simulink model "Hibrida_ultima"  (R2021b)
settings: Solver=VariableStepAuto  StartTime=0.0  StopTime=10.0  RelTol=1e-3
PreLoadFcn:
  | Fs = 44100;
  | f_tono = 500;
  | L = 32;
InitFcn:
  | Fs = 44100;
  | f_tono = 500;
  | L = 32;
undefined symbols (not defined in the file or in its folder): SzEstimado
settings Model: Creator=Vale Oieni  LastModifiedBy=ValeOieni

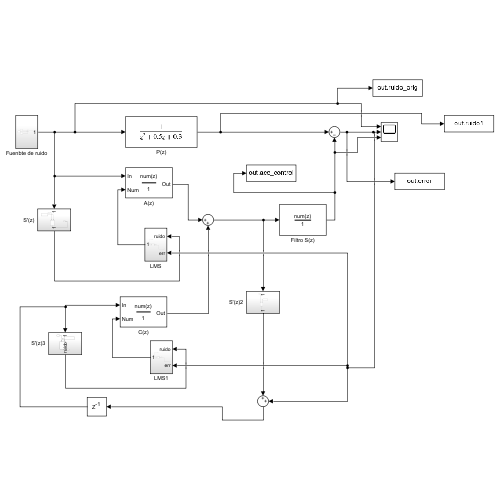
[thumbnail: Simulink's stored preview of the top-level diagram]
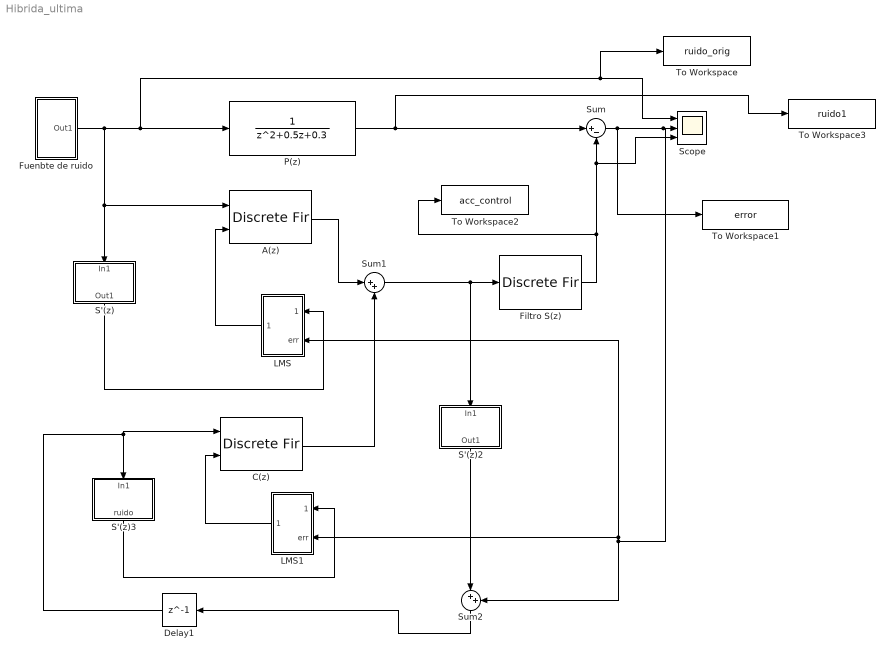
== system Hibrida_ultima ==
  A(z) : DiscreteFir  CoefSource=Input port  SampleTime=1/Fs
      settings: InputPortMap=u0,u1
  C(z) : DiscreteFir  CoefSource=Input port  SampleTime=1/Fs
      settings: InputPortMap=u0,u1
  Delay1 : Delay  DelayLength=1  InitialCondition=0
  Filtro S(z) : DiscreteFir  Coefficients=[0 0 -.5 .5 -.3 .2 -.1 .5 -.5]  InputProcessing=Columns as channels (frame based)  SampleTime=1/Fs
  Fuenbte de ruido : Subsystem
  LMS : Subsystem
  LMS1 : Subsystem
  P(z) : DiscreteTransferFcn  Denominator="[1 0.5  0.3]"
  S'(z) : Subsystem
  S'(z)2 : Subsystem
  S'(z)3 : Subsystem
  Scope : Scope  NumInputPorts=3
  Sum : Sum  Inputs=|+-
  Sum1 : Sum  Inputs=|++
  Sum2 : Sum  Inputs=|++
  To Workspace : ToWorkspace  VariableName=ruido_orig  SampleTime=-1
      settings: Save2DSignal=2-D array (concatenate along first dimension)
  To Workspace1 : ToWorkspace  VariableName=error  SampleTime=-1
      settings: Save2DSignal=2-D array (concatenate along first dimension)
  To Workspace2 : ToWorkspace  VariableName=acc_control  SampleTime=-1
      settings: Save2DSignal=2-D array (concatenate along first dimension)
  To Workspace3 : ToWorkspace  VariableName=ruido1  SampleTime=-1
      settings: Save2DSignal=2-D array (concatenate along first dimension)
  wires:
  Fuenbte de ruido/1(Out1) -> To Workspace/1, Scope/1, P(z)/1, A(z)/1, S'(z)/1(In1)
  P(z)/1 -> To Workspace3/1, Sum/1
  Filtro S(z)/1 -> Scope/3, Sum/2, To Workspace2/1
  Sum/1 -> To Workspace1/1, LMS1/2(err), LMS/2(err), Sum2/2, Scope/2
  Sum1/1 -> Filtro S(z)/1, S'(z)2/1(In1)
  A(z)/1 -> Sum1/1
  C(z)/1 -> Sum1/2
  LMS/1(Out1) -> A(z)/2
  LMS1/1(Out1) -> C(z)/2
  Sum2/1 -> Delay1/1
  S'(z)3/1(ruido) -> LMS1/1(ruido)
  S'(z)/1(Out1) -> LMS/1(ruido)
  S'(z)2/1(Out1) -> Sum2/1
  Delay1/1 -> C(z)/1, S'(z)3/1(In1)

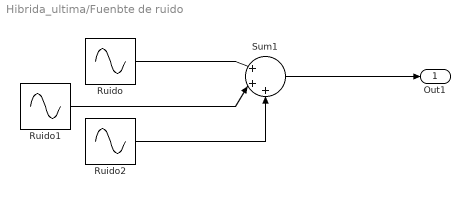
== system Hibrida_ultima/Fuenbte de ruido ==
  Ruido : Sin  Frequency=f_tono*(2*pi)  SampleTime=1/Fs
  Ruido1 : Sin  Frequency=2*f_tono*(2*pi)  SampleTime=1/Fs
  Ruido2 : Sin  Amplitude=2  Frequency=0.3*f_tono*(2*pi)  SampleTime=1/Fs
  Sum1 : Sum  Inputs=|+++
  Out1 : Outport
  wires:
  Ruido1/1 -> Sum1/2
  Sum1/1 -> Out1/1
  Ruido/1 -> Sum1/1
  Ruido2/1 -> Sum1/3

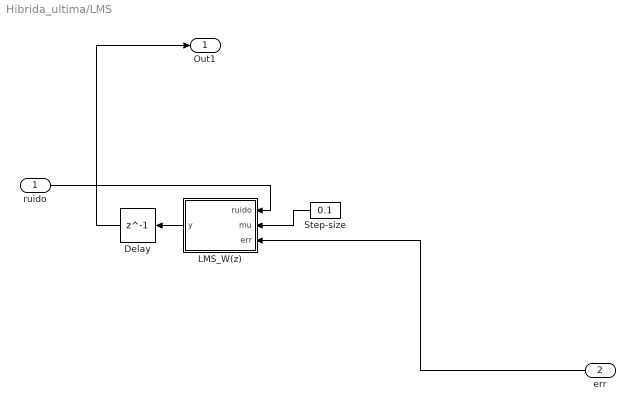
== system Hibrida_ultima/LMS ==
  ruido : Inport
  err : Inport  Port=2
  Delay : Delay  DelayLength=1  InitialCondition=0
  LMS_W(z) : MATLAB Function  TreatAsAtomicUnit=on
  Step-size : Constant  Value=0.1  SampleTime=1/Fs
  Out1 : Outport
  wires:
  LMS_W(z)/1(y) -> Delay/1
  Delay/1 -> Out1/1
  err/1 -> LMS_W(z)/3(err)
  Step-size/1 -> LMS_W(z)/2(mu)
  ruido/1 -> LMS_W(z)/1(ruido)

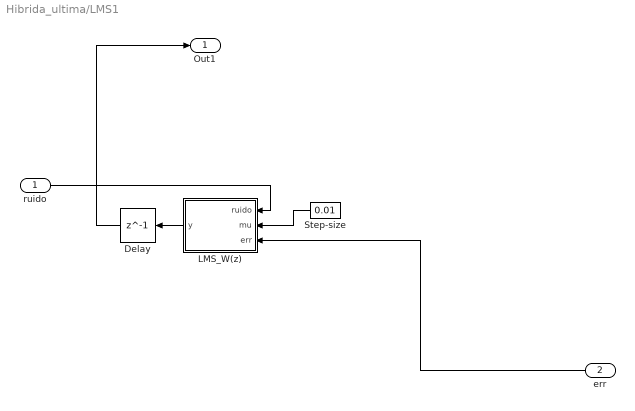
== system Hibrida_ultima/LMS1 ==
  ruido : Inport
  err : Inport  Port=2
  Delay : Delay  DelayLength=1  InitialCondition=0
  LMS_W(z) : MATLAB Function  TreatAsAtomicUnit=on
  Step-size : Constant  Value=0.01  SampleTime=1/Fs
  Out1 : Outport
  wires:
  ruido/1 -> LMS_W(z)/1(ruido)
  Step-size/1 -> LMS_W(z)/2(mu)
  err/1 -> LMS_W(z)/3(err)
  Delay/1 -> Out1/1
  LMS_W(z)/1(y) -> Delay/1

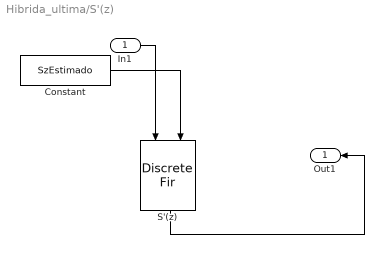
== system Hibrida_ultima/S'(z) ==
  In1 : Inport
  Constant : Constant  Value=SzEstimado  SampleTime=1/Fs
  S'(z) : DiscreteFir  CoefSource=Input port  SampleTime=1/Fs
      settings: InputPortMap=u0,u1
  Out1 : Outport
  wires:
  Constant/1 -> S'(z)/2
  In1/1 -> S'(z)/1
  S'(z)/1 -> Out1/1

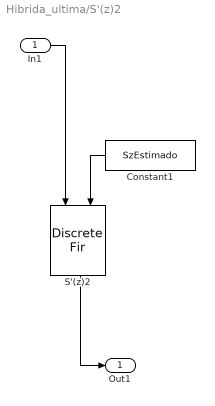
== system Hibrida_ultima/S'(z)2 ==
  In1 : Inport
  Constant1 : Constant  Value=SzEstimado  SampleTime=1/Fs
  S'(z)2 : DiscreteFir  CoefSource=Input port  SampleTime=1/Fs
      settings: InputPortMap=u0,u1
  Out1 : Outport
  wires:
  In1/1 -> S'(z)2/1
  Constant1/1 -> S'(z)2/2
  S'(z)2/1 -> Out1/1

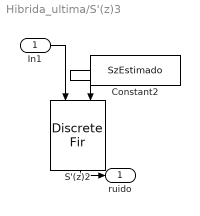
== system Hibrida_ultima/S'(z)3 ==
  In1 : Inport
  Constant2 : Constant  Value=SzEstimado  SampleTime=1/Fs
  S'(z)2 : DiscreteFir  CoefSource=Input port  SampleTime=1/Fs
      settings: InputPortMap=u0,u1
  ruido : Outport
  wires:
  Constant2/1 -> S'(z)2/2
  In1/1 -> S'(z)2/1
  S'(z)2/1 -> ruido/1

== matlab function Hibrida_ultima/LMS1/LMS_W(z) ==
  data: ruido input; mu input; y output; err input
function y = fcn(ruido, mu, err)
    L = 32;
    %Pesos w_n
    persistent w_n
    if isempty(w_n)
        w_n = zeros(1, L); % inicializa w en cero, largo L
    end
    %Vector de ruido
    persistent x
    if isempty(x)
        x = zeros(1, L); % inicializa x en cero, largo L
    end
    %Vaciado de x
    x(2:L) = x(1:L-1);
    x(1) = ruido;
    %Actualizacion
    xvar = x;
    w = w_n;
    w = w + mu*err*xvar;   
    w_n = w;
    %Asignación a la salida
    y = w;
end

== matlab function Hibrida_ultima/LMS/LMS_W(z) ==
  data: ruido input; mu input; y output; err input
function y = fcn(ruido, mu, err)
    L = 32;
    %Pesos w_n
    persistent w_n
    if isempty(w_n)
        w_n = zeros(1, L); % inicializa w en cero, largo L
    end
    %Vector de ruido
    persistent x
    if isempty(x)
        x = zeros(1, L); % inicializa x en cero, largo L
    end
    %Vaciado de x
    x(2:L) = x(1:L-1);
    x(1) = ruido;
    %Actualizacion
    xvar = x;
    w = w_n;
    w = w + mu*err*xvar;   
    w_n = w;
    %Asignación a la salida
    y = w;
end
